simulink library "Lab_b"  (R2023b)
settings: Solver=VariableStepAuto  StartTime=0.0  StopTime=10.0  RelTol=1e-3
values from neighbouring files (symbols this model uses):
  Bm = 0.006126    [parameters.m]
  J = 0.1646    [parameters.m]
  ke = 1.8    [parameters.m]
  kt = 1.8    [parameters.m]
  La = 0.002012    [parameters.m]
undefined symbols (not defined in the file or in its folder): ra
libraries: fl_lib x11, nesl_utility x5, spsControlledVoltageSourceLib x1, spsDCMachineLib x1, simulink x1
settings Model: Creator=Student  LastModifiedBy=Student

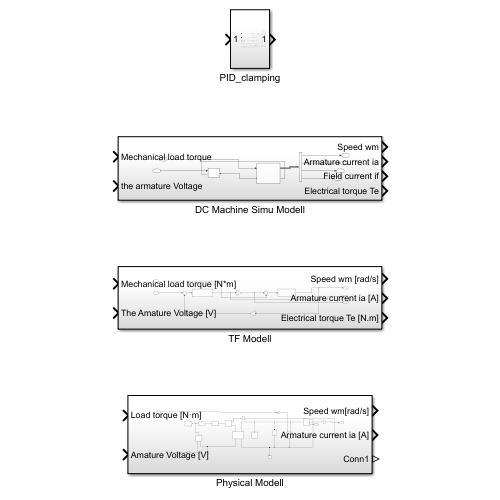
[thumbnail: Simulink's stored preview of the top-level diagram]
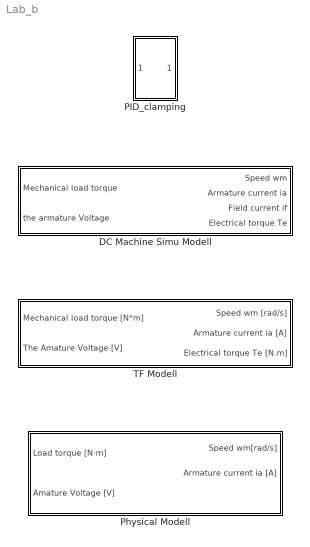
== system Lab_b ==
  DC Machine Simu Modell : Subsystem
  PID_clamping : Subsystem
  Physical Modell : Subsystem
  TF Modell : Subsystem

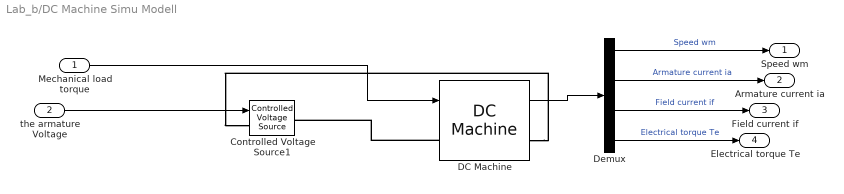
== system Lab_b/DC Machine Simu Modell ==
  Mechanical load torque : Inport
  the armature Voltage : Inport  Port=2
  Controlled Voltage Source1 : spsControlledVoltageSourceLib/Controlled Voltage Source  Initialize=on  Source_Type=DC  Amplitude=0  Phase=0  Frequency=0  Measurements=None
  DC Machine : spsDCMachineLib/DC Machine  PresetModel=No  MechanicalLoad=Torque TL  FieldType=Permanent magnet  ShowDetailedParameters=on  MeasurementBus=off  RLa="[ 0.1514  0.002012]"  RLf="[ 240  120]"  Laf=1.8  MachineConstant=Torque constant (N.m/A)  Ke=1.8  Kt=1.8  J=0.1646  Bm=0.006126  Tf=0  w0=0  Ifinit=1  TsPowergui=0  TsBlock=-1
  Demux : Demux
  Speed wm : Outport
  Armature current ia : Outport  Port=2
  Field current if : Outport  Port=3
  Electrical torque Te : Outport  Port=4
  wires:
  Mechanical load torque/1 -> DC Machine/1
  DC Machine/1 -> Demux/1
  Demux/4 -> Electrical torque Te/1  "Electrical torque Te"
  the armature Voltage/1 -> Controlled Voltage Source1/1
  Demux/2 -> Armature current ia/1  "Armature current ia"
  Demux/1 -> Speed wm/1  "Speed wm"
  Demux/3 -> Field current if/1  "Field current if"
  connections:
  DC Machine/LConn1 -- Controlled Voltage Source1/RConn1
  DC Machine/RConn1 -- Controlled Voltage Source1/LConn1

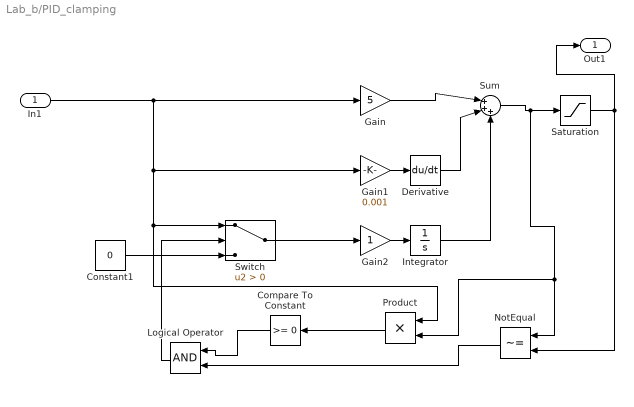
== system Lab_b/PID_clamping ==
  In1 : Inport
  Compare To Constant : simulink/Logic and Bit Operations/Compare To Constant  relop=>=  const=0  OutDataTypeStr=boolean
  Constant1 : Constant  Value=0
  Derivative : Derivative
  Gain : Gain  Gain=5
  Gain1 : Gain  Gain=0.001
  Gain2 : Gain
  Integrator : Integrator
  Logical Operator : Logic  AllPortsSameDT=off  OutDataTypeStr=boolean
  NotEqual : RelationalOperator  Operator=~=  OutDataTypeStr=boolean  RndMeth=Simplest  InputSameDT=off
  Product : Product
  Saturation : Saturate  UpperLimit=500  LowerLimit=-500
  Sum : Sum  Inputs=|+++
  Switch : Switch  Criteria=u2 > Threshold  SaturateOnIntegerOverflow=off  InputSameDT=off
  Out1 : Outport
  wires:
  Derivative/1 -> Sum/2
  Gain2/1 -> Integrator/1
  Switch/1 -> Gain2/1
  Sum/1 -> Product/2, NotEqual/1, Saturation/1
  Gain1/1 -> Derivative/1
  Integrator/1 -> Sum/3
  Saturation/1 -> Out1/1, NotEqual/2
  Logical Operator/1 -> Switch/2
  In1/1 -> Switch/1, Product/1, Gain1/1, Gain/1
  Product/1 -> Compare To Constant/1
  NotEqual/1 -> Logical Operator/2
  Compare To Constant/1 -> Logical Operator/1
  Constant1/1 -> Switch/3
  Gain/1 -> Sum/1

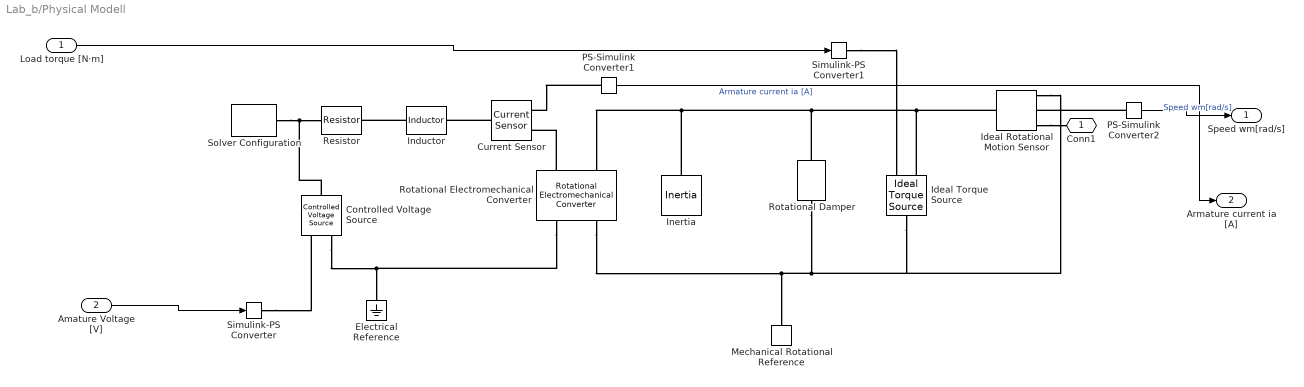
== system Lab_b/Physical Modell ==
  Load torque [N·m] : Inport
  Amature Voltage [V] : Inport  Port=2
  Controlled Voltage Source : fl_lib/Electrical/Electrical Sources/Controlled Voltage Source
  Current Sensor : fl_lib/Electrical/Electrical Sensors/Current Sensor
  Electrical Reference : fl_lib/Electrical/Electrical Elements/Electrical Reference
  Ideal Rotational Motion Sensor : fl_lib/Mechanical/Mechanical Sensors/Ideal Rotational Motion Sensor  reference=foundation.enum.MeasurementReference.difference  acceleration_port=false  velocity_port=true  position_port=true  wrap_angle=false  offset=0 rad
  Ideal Torque Source : fl_lib/Mechanical/Mechanical Sources/Ideal Torque Source
  Inductor : fl_lib/Electrical/Electrical Elements/Inductor  l=La H  r=0 Ohm  g=1e-9 1/Ohm  i_specify=off  i_priority=None  i=0 A  i_nominal_specify=off  i_nominal_unit=A  i_nominal_value=1  v_specify=off  v_priority=None  v=0 V  v_nominal_specify=off  v_nominal_unit=V  v_nominal_value=1  i_L_specify=off  i_L_priority=High  i_L=0 A  i_L_nominal_specify=off  i_L_nominal_unit=A  i_L_nominal_value=1
  Inertia : fl_lib/Mechanical/Rotational Elements/Inertia  inertia=J kg*m^2  num_ports=foundation.enum.numPorts2.one  w_specify=off  w_priority=High  w=0 rad/s  w_nominal_specify=off  w_nominal_unit=rad/s  w_nominal_value=1  t_specify=off  t_priority=None  t=0 N*m  t_nominal_specify=off  t_nominal_unit=N*m  t_nominal_value=1
  Mechanical Rotational Reference : fl_lib/Mechanical/Rotational Elements/Mechanical Rotational Reference
  PS-Simulink Converter1 : nesl_utility/PS-Simulink Converter  PhysicalDomain=network_engine_domain  SubClassName=ps_output  LeftPortType=input  RightPortType=output  PseudoPeriodic=off  Frequencies=[]  VectorFormat=inherit  Unit=inherit  AffineConversion=off
  PS-Simulink Converter2 : nesl_utility/PS-Simulink Converter  PhysicalDomain=network_engine_domain  SubClassName=ps_output  LeftPortType=input  RightPortType=output  PseudoPeriodic=off  Frequencies=[]  VectorFormat=inherit  Unit=inherit  AffineConversion=off
  Resistor : fl_lib/Electrical/Electrical Elements/Resistor  R=ra Ohm  i_specify=off  i_priority=None  i=0 A  i_nominal_specify=off  i_nominal_unit=A  i_nominal_value=1  v_specify=off  v_priority=None  v=0 V  v_nominal_specify=off  v_nominal_unit=V  v_nominal_value=1
  Rotational Electromechanical Converter : fl_lib/Electrical/Electrical Elements/Rotational Electromechanical Converter  K=ke V*s/rad  i_specify=off  i_priority=None  i=0 A  i_nominal_specify=off  i_nominal_unit=A  i_nominal_value=1  v_specify=off  v_priority=None  v=0 V  v_nominal_specify=off  v_nominal_unit=V  v_nominal_value=1  t_specify=off  t_priority=None  t=0 N*m  t_nominal_specify=off  t_nominal_unit=N*m  t_nominal_value=1  w_specify=off  w_priority=None  w=0 rad/s  w_nominal_specify=off  w_nominal_unit=rad/s  w_nominal_value=1
  Rotational Damper : fl_lib/Mechanical/Rotational Elements/Rotational Damper  D=Bm N*m*s/rad  w_specify=off  w_priority=None  w=0 rad/s  w_nominal_specify=off  w_nominal_unit=rad/s  w_nominal_value=1  t_specify=off  t_priority=None  t=0 N*m  t_nominal_specify=off  t_nominal_unit=N*m  t_nominal_value=1
  Simulink-PS Converter : nesl_utility/Simulink-PS Converter  PhysicalDomain=network_engine_domain  SubClassName=ps_input  LeftPortType=input  RightPortType=output  PseudoPeriodic=off  Frequencies=[]  NoiseDistribution=none  NoiseParameters=[]  Unit=1  AffineConversion=off  FilteringAndDerivatives=provide  SimscapeFilterOrder=1  InputFilterTimeConstant=0.001  UdotUserProvided=0
  Simulink-PS Converter1 : nesl_utility/Simulink-PS Converter  PhysicalDomain=network_engine_domain  SubClassName=ps_input  LeftPortType=input  RightPortType=output  PseudoPeriodic=off  Frequencies=[]  NoiseDistribution=none  NoiseParameters=[]  Unit=1  AffineConversion=off  FilteringAndDerivatives=provide  SimscapeFilterOrder=1  InputFilterTimeConstant=0.001  UdotUserProvided=0
  Solver Configuration : nesl_utility/Solver Configuration  PhysicalDomain=network_engine_domain  SubClassName=solver  LeftPortType=input  RightPortType=generic  Tones=[]  Harmonics=[]  SimulateNoise=off  Profile=off  UseLocalSampling=off  EnableSwitchedLinearOptims=on  FrequencyDomain=off  UseCCode=off  RelTol=0.001  AbsTol=0.001  MinStep=1e-09  ToWorkspace=off  RevertToSquareIcSolve=off  NumHomotopyIterations=100  PhasorMode=off  PhasorModeNumHarmonics=1  ConsistencySolver=NEWTON_XTOL_AFTER_FTOL  IndexReductionMethod=DerivativeReplacement  DoDC=off  ResidualTolerance=1e-09  ConsistencyTolSource=GLOBAL  ConsistencyAbsTol=0.001  ConsistencyRelTol=0.001  ConsistencyTolFactor=0.001  UseLocalSolver=off  LocalSolverChoice=NE_BACKWARD_EULER_ADVANCER  ResolveIndetEquations=on  FunctionEvalNumThread=1  LocalSolverSampleTime=0.001  DoFixedCost=off  MaxNonlinIter=3  MaxModeIter=2  ComputeImpulses=off  ImpulseIterations=2  LinearAlgebra=auto  LinearAlgebraNumThread=0  EquationFormulation=NE_TIME_EF  DelaysMemoryBudget=1024  AutomaticFiltering=on  FilteringTimeConstant=0.001  PartitionStorageMethod=AS_NEEDED  PartitionMemoryBudget=1024  PartitionMethod=ROBUST  MultibodyUseLocalSolver=off  MultibodyLocalSolverChoice=ODE1  MultibodyLocalSolverSampleTime=0.001
  Conn1 : PMIOPort  Side=Right
  Speed wm[rad/s] : Outport
  Armature current ia [A] : Outport  Port=2
  wires:
  Load torque [N·m]/1 -> Simulink-PS Converter1/1
  PS-Simulink Converter1/1 -> Armature current ia [A]/1  "Armature current ia [A]"
  Amature Voltage [V]/1 -> Simulink-PS Converter/1
  PS-Simulink Converter2/1 -> Speed wm[rad/s]/1  "Speed wm[rad/s]"
  connections:
  PS-Simulink Converter2/LConn1 -- Ideal Rotational Motion Sensor/RConn2
  Ideal Rotational Motion Sensor/LConn1 -- Ideal Torque Source/RConn2 -- Rotational Damper/LConn1 -- Inertia/LConn1 -- Rotational Electromechanical Converter/LConn2
  Rotational Electromechanical Converter/RConn2 -- Rotational Damper/RConn1 -- Ideal Torque Source/LConn1 -- Ideal Rotational Motion Sensor/RConn1 -- Mechanical Rotational Reference/LConn1
  Solver Configuration/RConn1 -- Controlled Voltage Source/LConn1 -- Resistor/LConn1
  Controlled Voltage Source/RConn2 -- Rotational Electromechanical Converter/RConn1 -- Electrical Reference/LConn1
  Ideal Rotational Motion Sensor/RConn3 -- Conn1/RConn1
  Rotational Electromechanical Converter/LConn1 -- Current Sensor/RConn2
  PS-Simulink Converter1/LConn1 -- Current Sensor/RConn1
  Current Sensor/LConn1 -- Inductor/RConn1
  Simulink-PS Converter/RConn1 -- Controlled Voltage Source/RConn1
  Simulink-PS Converter1/RConn1 -- Ideal Torque Source/RConn1
  Inductor/LConn1 -- Resistor/RConn1

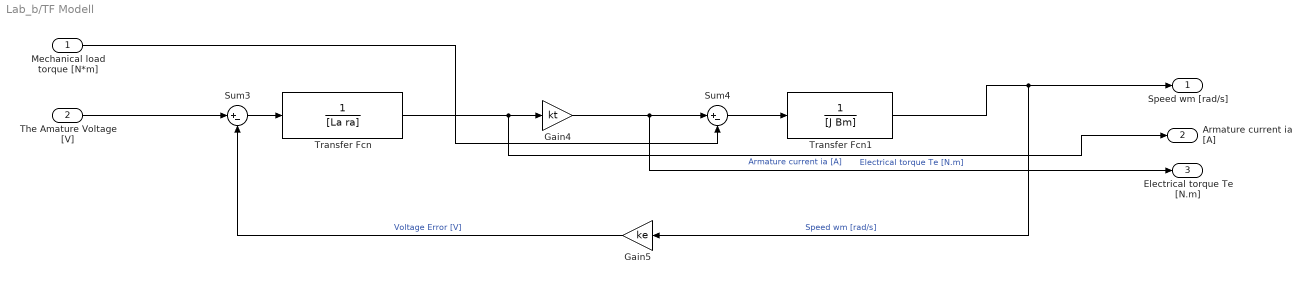
== system Lab_b/TF Modell ==
  Mechanical load torque [N*m] : Inport
  The Amature Voltage [V] : Inport  Port=2
  Gain4 : Gain  Gain=kt
  Gain5 : Gain  Gain=ke
  Sum3 : Sum  Inputs=|+-
  Sum4 : Sum  Inputs=|+-
  Transfer Fcn : TransferFcn  Denominator=[La ra]
  Transfer Fcn1 : TransferFcn  Denominator=[J Bm]
  Speed wm [rad/s] : Outport
  Armature current ia [A] : Outport  Port=2
  Electrical torque Te [N.m] : Outport  Port=3
  wires:
  Sum4/1 -> Transfer Fcn1/1
  Gain4/1 -> Electrical torque Te [N.m]/1, Sum4/1  "Electrical torque Te [N.m]"
  Sum3/1 -> Transfer Fcn/1
  Transfer Fcn/1 -> Armature current ia [A]/1, Gain4/1  "Armature current ia [A]"
  Transfer Fcn1/1 -> Speed wm [rad/s]/1, Gain5/1  "Speed wm [rad/s]"
  The Amature Voltage [V]/1 -> Sum3/1
  Gain5/1 -> Sum3/2  "Voltage Error [V]"
  Mechanical load torque [N*m]/1 -> Sum4/2
